simulink model "mu_t_2021b_temp"  (R2023b)
settings: Solver=VariableStepAuto  StartTime=0.0  StopTime=120  FixedStep=0.01  RelTol=1e-3
InitFcn:
  | %rho_0t=[0.29;0.29;0.29]; %m
  | %V_0t=[-0.001;-0.001;0];%[-0.0005;-0.0005;0];
  | %w_t=[0;0;-0.002];
  | 
  | 
  | %rho_0t=[0.3;0.3;0.2]; %m
  | %V_0t=[-0.001;-0.001;0];%[-0.0005;-0.0005;0];
  | %w_t=[0;0;-0.001];
values from neighbouring files (symbols this model uses):
  g_cm = zeros(4,4,n)    [Initiate_KUKA_inv.m]    (also in KUKA_Main.m)
  iota0 = eye(6,6)    [Initiate_KUKA_inv.m]    (also in KUKA_Main.m)
  K_d = 10*[1.3*eye(3) zeros(3);zeros(3) 0.8*eye(3)]    [Initiate_FQ.m]    (also in Initiate_KUKA_inv.m = 5*[0.7*eye(3) zeros(3);zeros(3) 0.5*eye(3)]; KUKA_Main.m = 50*[0.7*eye(3) zeros(3);zeros(3) 0.5*eye(3)])
  K_i = 5*[0.1*eye(3) zeros(3);zeros(3) 0.01*eye(3)]    [Initiate_FQ.m]    (also in Initiate_KUKA_inv.m = 5*[0.01*eye(3) zeros(3);zeros(3) 0.001*eye(3)]; KUKA_Main.m = 50*[0.01*eye(3) zeros(3);zeros(3) 0.001*eye(3)])
  K_p = 100*[0.1 0 0 0 0 0;0 0.1 0 0 0 0; 0 0 0.1 0 0 0; 0 0 0 0.01 0 0 ... (first row only)    [Initiate_FQ.m]    (also in Initiate_KUKA_inv.m = 5*[0.1 0 0 0 0 0;0 0.1 0 0 0 0; 0 0 0.1 0 0 0; 0 0 0 0.01 0 ; KUKA_Main.m = 50*[0.1 0 0 0 0 0;0 0.1 0 0 0 0; 0 0 0.1 0 0 0; 0 0 0 0.01 0)
  K_w = 200*eye(7)    [Initiate_FQ.m]
  K_wd = 2*eye(7)    [Initiate_FQ.m]
  M0 = M_temp.M0.data(:,:,1)    [Initiate_FQ.m]    (also in KUKA_Main.m)
  m0 = robot.Bodies{1,n+1}.Mass    [Initiate_KUKA_inv.m]    (also in KUKA_Main.m)
  m0_frak = diag_M(1:6,1:6)    [Initiate_KUKA_inv.m]
  M0m = M_temp.M0m.data(:,:,1)    [Initiate_FQ.m]    (also in KUKA_Main.m)
  m_diag = diag_M(7:end,7:end)    [Initiate_KUKA_inv.m]
  M_t = (((Adjoint(g_It))'\M_t_body)/(Adjoint(g_It)))    [Initiate_FQ.m]    (also in Initiate_KUKA_inv.m = [eye(3)*mt zeros(3); zeros(3) eye(3)*80]; KUKA_Main.m = [eye(3)*mt zeros(3); zeros(3) eye(3)*80])
  Mm = simplify(transpose(Xi_m)*transpose(Lm)*diagM*Lm*Xi_m)    [KUKA_Main.m]
  mm = zeros(1,n)    [Initiate_KUKA_inv.m]    (also in KUKA_Main.m)
  mu = P0    [Initiate_FQ.m]    (also in Initiate_KUKA_inv.m = zeros(6,1); KUKA_Main.m = P)
  mu_t = inv((Adjoint(g_It))')*M_t_body*[V_It;w_t]    [Initiate_FQ.m]    (also in Initiate_KUKA_inv.m = M_t*[V_0t;w_t]; KUKA_Main.m = M_t*[V_0t;w_t])
  q_dot_m = [0;0;0;0;0;0;0]    [Initiate_FQ.m]    (also in Initiate_KUKA_inv.m; KUKA_Main.m = [qdot1;qdot2;qdot3;qdot4;qdot5;qdot6;qdot7])
  q_m = [0.2;1.2;0.3;2.5;0.5;1.5;0.6]    [Initiate_FQ.m]    (also in Initiate_KUKA_inv.m = [0;0;0;0;0;0;0]; KUKA_Main.m = [q_m1;q_m2;q_m3;q_m4;q_m5;q_m6;q_m7])
  rho_It = [-0.3;-0.3;-0.1]    [Initiate_FQ.m]
  sc_size = 1    [Initiate_KUKA_inv.m]    (also in KUKA_Main.m)
  V_I0 = [-0.0001;-0.0001;0.0;-0.001;0.001;0.002]    [Initiate_FQ.m]    (also in Initiate_KUKA_inv.m = [0;0;0;0;0;0]; KUKA_Main.m = [0;0;0;0;0;0])
  V_It = 0.1.*[0.01;0.01;0]    [Initiate_FQ.m]
  Xi_m = Xi_m(1:robot.n*6,1:robot.n)    [KUKA_Main.m]
  Xi_m_matrix = zeros(6*n,n)    [Initiate_KUKA_inv.m]    (also in KUKA_Main.m)
undefined symbols (not defined in the file or in its folder): Dt, Dt_s, g_cm0, g_It00, I0, Ie, Im, me, noise_st, X, Y, Z
libraries: nesl_utility x195, sm_lib x180, robotcorelib x12, simulink x6
(part 1 of 8)
settings Model: Creator=Bmmog  LastModifiedBy=Bmmog
settings SolverCC: ZeroCrossAlgorithm=Adaptive
settings DataIOCC: ReturnWorkspaceOutputsName=tp1ae71780_9f9b_41fc_80d6_93119145c185
settings DebuggingCC: UnconnectedInputMsg=warning  UnconnectedOutputMsg=warning  UnconnectedLineMsg=warning
settings ModelReferenceCC: EnableRefExpFcnMdlSchedulingChecks=on
settings RTWCC: DLArmComputeVersion=19.05
settings ExplorerConfigSet: InternalSimMechanicsExplorerSettings="<ExplorerConfiguration><canonicalview>default</canonicalview><AnimationSetting><BasePlaybackSpeed>1.0</BasePlaybackSpeed><PlaybackSpeedFactor>1.0</PlaybackSpeedFactor></AnimationSetting><TilePanel><TileInfo><Tiles Columns=\"1\" Count=\"1\" Rows=\"1\"><Column Weight=\"1\"/><Row Weight=\"1\"/><Tile Height=\"1\" Width=\"1\" X=\"0\" Y=\"0\"/></Tiles></TileInfo><SceneInfo><SceneViewer><BGColor><R>0.60000002384185791</R><G>0.60000002384185791</G><B>0.60000002384185791</B></BGColor><Camera><DoPerspective>off</DoPerspective><Position><X>0.589775080981291833</X><Y>-1.46493128404912909</Y><Z>0.784080153206962893</Z></Position><Center><X>-0.149105792545367294</X><Y>0.231974603355053599</Y><Z>-0.0696143327165401893</Z></Center><Up><X>0.0771327039681207333</X><Y>0.474680075340175867</Y><Z>0.876772132343182631</Z></Up><ViewLimDist>1</ViewLimDist><YLim>0.0938244390560590141</YLim><XLim>0.109167654126007874</XLim></Camera></SceneViewer></SceneInfo></TilePanel><MechEditorPanel><Cameras/><GfxPanelCameraMap/><VideoCreator><PlaybackSpeedRatio>1.0</PlaybackSpeedRatio><FrameRate>30</FrameRate><VideoFormat>Motion JPEG AVI</VideoFormat><FrameSize>auto</FrameSize></VideoCreator></MechEditorPanel></ExplorerConfiguration>"

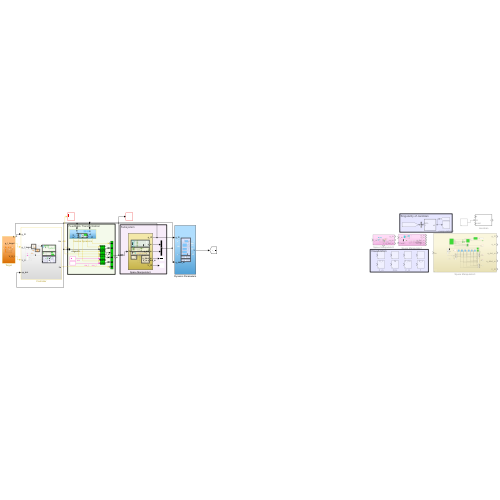
[thumbnail: Simulink's stored preview of the top-level diagram]
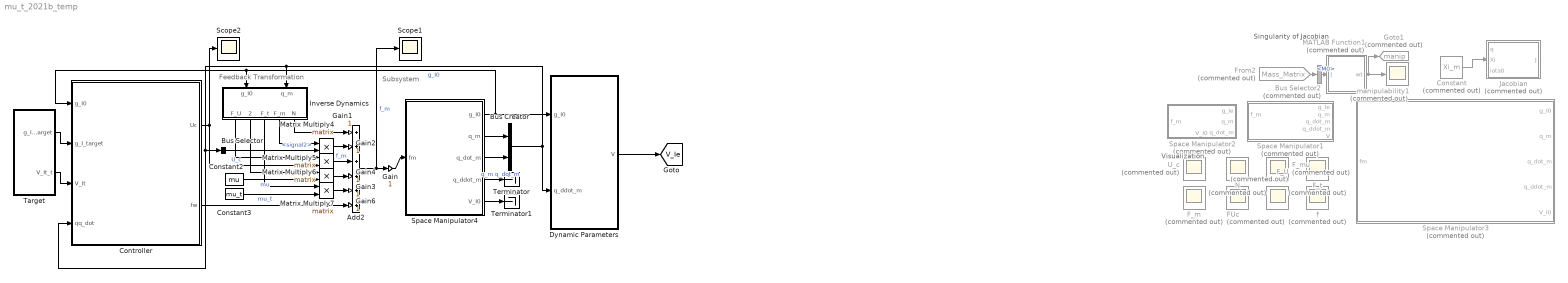
== system mu_t_2021b_temp ==
  note: Subsystem
  note: Feedback Transformation
  note: Singularity of Jacobian
  note: Visualization
  Add2 : Sum  Inputs=++++++
  Bus Creator : BusCreator  Inputs=2
  Bus Selector : BusSelector  OutputSignals=signal2
  Bus Selector2 : BusSelector  Commented=on  OutputSignals=M0
  Constant : Constant  Commented=on  Value=Xi_m
  Constant2 : Constant  Value=mu
  Constant3 : Constant  Value=mu_t
  Controller : Subsystem
  Dynamic Parameters : Subsystem
  FUc : Scope  Commented=on
  F_U : Scope  Commented=on
  F_m : Scope  Commented=on
  F_mu : Scope  Commented=on
  F_t : Scope  Commented=on
  From2 : From  Commented=on  GotoTag=Mass_Matrix  TagVisibility=global
  Gain{,1..4,6} (6 alike) : Gain
  Goto1 : Goto  Commented=on  GotoTag=manip  TagVisibility=global
  Inverse Dynamics : Subsystem
  Jacobian : MATLAB Function  Commented=on  TreatAsAtomicUnit=on
  MATLAB Function1 : MATLAB Function  Commented=on  TreatAsAtomicUnit=on
  Matrix Multiply{4..7} (4 alike) : Product  Multiplication=Matrix(*)
  N : Scope  Commented=on
  Scope1 : Scope
  Scope2 : Scope
  Space Manipulator1 : Subsystem  Commented=on
  Space Manipulator2 : Subsystem  Commented=on
      settings: PortSchema="{\"entries\":[{\"content\":{\"sides\":[{\"content\":{\"connectorIds\":[\"In1\"]},\"type\":\"ConnectorPlacement.EquallySpacedRectSide\",\"uuid\":\"530c21f8-fd54-4a84-9ce8-3a95f84fd0bc\"},{\"content\":{\"connectorIds\":[\"Out1\",\"Out2\",\"Out3\"],\"side\":\"RIGHT\"},\"type\":\"ConnectorPlacement.EquallySpacedRectSide\",\"uuid\":\"3d1ca3bb-457e-45f0-8a55-d4d08374b273\"},{\"content\":{\"connectorIds\":[],\"side\":\"TOP\"},\"type\":\"ConnectorPlacement.EquallySpacedRectSide\",\"uuid\":\"24d553c5-4913-4f02-8b85-43cdd650a04b\"},{\"content\":{\"connectorIds\":[\"Out4\"],\"side\":\"BOTTOM\"},\"type\":\"ConnectorPlacement.EquallySpacedRectSide\",\"uuid\":\"b0ec554d-8dce-4af2-8e04-261e5fffea9f\"}]},\"type\":\"ConnectorPlacement.EquallySpacedConnector\",\"uuid\":\"032cf2d7-4a61-467d-a02b-78dcb243a1bb\"}],\"packageUris\":[\"http://schema.mathworks.com/mf0/Connector/R2020b\"],\"version\":\"1.0\"}"
  Space Manipulator3 : Subsystem  Commented=on
  Space Manipulator4 : Subsystem
  Target : Subsystem
  Terminator : Terminator
  Terminator1 : Terminator
  U_c : Scope  Commented=on
  f : Scope  Commented=on
  manipulability1 : Scope  Commented=on
  tag scope: V_Ie=global
  wires:
  Target/2(V_It_t) -> Controller/3(V_It)
  Space Manipulator4/1(g_I0) -> Inverse Dynamics/1(g_I0), Controller/1(g_I0), Dynamic Parameters/1(g_I0)  "g_I0"
  Inverse Dynamics/3(F_t) -> Matrix Multiply7/1
  Matrix Multiply5/1 -> Add2/3  "f_m"
  Inverse Dynamics/2(F_mu) -> Matrix Multiply6/1
  Inverse Dynamics/4(F_m) -> Matrix Multiply4/1
  Constant3/1 -> Matrix Multiply7/2  "mu_t"
  Constant2/1 -> Matrix Multiply6/2  "mu"
  Bus Creator/1 -> Inverse Dynamics/2("q_m "), Bus Selector/1, Controller/4(qq_dot), Dynamic Parameters/2(q_ddot_m)
  Bus Selector/1 -> Matrix Multiply4/2  "<signal2>"
  Space Manipulator4/4(q_ddot_m) -> Terminator/1  "q_m q_dot_m"
  Gain/1 -> Space Manipulator4/1(fm)
  Target/1(g_I_target) -> Controller/2(g_I_target)
  Add2/1 -> Scope1/1, Gain/1  "f_m"
  Gain1/1 -> Add2/1
  Gain2/1 -> Add2/2
  Gain3/1 -> Add2/5
  Gain4/1 -> Add2/4
  Controller/1(Uc) -> Scope2/1, Matrix Multiply5/2  "U_c"
  Inverse Dynamics/1(F_U) -> Matrix Multiply5/1
  Matrix Multiply4/1 -> Gain2/1
  Matrix Multiply6/1 -> Gain4/1
  Inverse Dynamics/5(N) -> Gain1/1
  Matrix Multiply7/1 -> Gain3/1
  Space Manipulator4/2(q_m) -> Bus Creator/1
  Space Manipulator4/3(q_dot_m) -> Bus Creator/2
  Space Manipulator4/5(V_I0) -> Terminator1/1
  Constant/1 -> Jacobian/2(Xi)
  From2/1 -> Bus Selector2/1
  Bus Selector2/1 -> MATLAB Function1/1(J)  "<M0>"
  Gain6/1 -> Add2/6
  MATLAB Function1/1(wt) -> Goto1/1, manipulability1/1
  Controller/2(fw) -> Gain6/1
  Dynamic Parameters/1(V) -> [V_Ie]

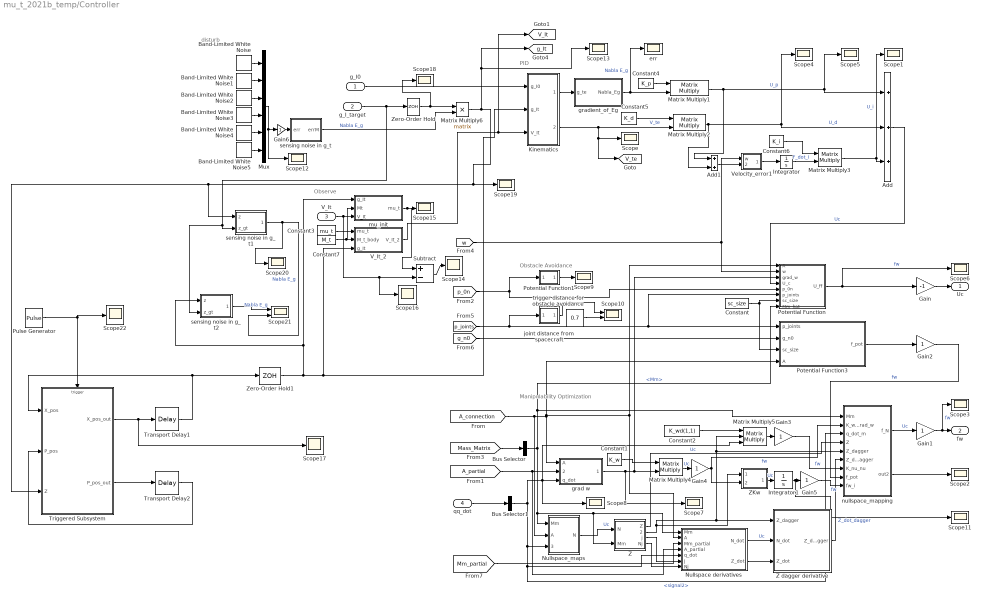
== system mu_t_2021b_temp/Controller ==
  note: PID
  note: Manipulability Optimization
  note: Obstacle Avoidance
  note: Observe
  note: disturb
  g_I0 : Inport
  g_I_target : Inport  Port=2
  V_It : Inport  Port=3
  qq_dot : Inport  Port=4
  Add : Sum  Inputs=+++
  Add1 : Sum
  Band-Limited White Noise : simulink/Sources/Band-Limited White Noise  Cov=[noise_st]  Ts=Dt_s  seed=[23341]
  Band-Limited White Noise1 : simulink/Sources/Band-Limited White Noise  Cov=[noise_st]  Ts=Dt_s  seed=[23342]
  Band-Limited White Noise2 : simulink/Sources/Band-Limited White Noise  Cov=[noise_st]  Ts=Dt_s  seed=[23343]
  Band-Limited White Noise3 : simulink/Sources/Band-Limited White Noise  Cov=[noise_st]  Ts=Dt_s  seed=[23344]
  Band-Limited White Noise4 : simulink/Sources/Band-Limited White Noise  Cov=[noise_st]  Ts=Dt_s  seed=[23345]
  Band-Limited White Noise5 : simulink/Sources/Band-Limited White Noise  Cov=[noise_st]  Ts=Dt_s  seed=[23346]
  Bus Selector : BusSelector  OutputSignals=Mm
  Bus Selector1 : BusSelector  OutputSignals=signal2
  Constant : Constant  Value=sc_size
  Constant1 : Constant  Value=K_w
  Constant2 : Constant  Value=K_wd(1,1)
  Constant3 : Constant  Value=mu_t
  Constant4 : Constant  Value=K_p
  Constant5 : Constant  Value=K_d
  Constant6 : Constant  Value=K_i
  Constant7 : Constant  Value=M_t
  Gain : Gain  Gain=-1
  Gain{1..6} (6 alike) : Gain
  Integrator : Integrator
  Integrator1 : Integrator
  Kinematics : Subsystem
  Matrix Multiply{1..4,6} (5 alike) : Product  Multiplication=Matrix(*)
  Matrix Multiply5 : Product  Inputs=3  Multiplication=Matrix(*)
  Mux : Mux  Inputs=6
  Nullspace derivatives : MATLAB Function  TreatAsAtomicUnit=on
  Nullspace_maps : MATLAB Function  TreatAsAtomicUnit=on
  Potential Function : MATLAB Function  TreatAsAtomicUnit=on
  Potential Function1 : MATLAB Function  TreatAsAtomicUnit=on
  Potential Function3 : MATLAB Function  TreatAsAtomicUnit=on
  Pulse Generator : DiscretePulseGenerator  PulseType=Time based  Period=Dt  PulseWidth=10
  Scope{,1..9,11..20,22} (21 alike) : Scope
  Scope10 : Scope  NumInputPorts=2
  Scope21 : Scope  NumInputPorts=2
  Subtract : Sum  Inputs=+-
  Transport Delay1 : TransportDelay  DelayTime=Dt  InitialOutput=g_It00  TransDelayFeedthrough=on
  Transport Delay2 : TransportDelay  DelayTime=Dt  InitialOutput=zeros(6)  TransDelayFeedthrough=on
  Triggered Subsystem : Subsystem  TreatAsAtomicUnit=on
  V_It_2 : MATLAB Function  TreatAsAtomicUnit=on
  Velocity_error1 : MATLAB Function  TreatAsAtomicUnit=on
  Z : MATLAB Function  TreatAsAtomicUnit=on
  Z dagger derivative : MATLAB Function  TreatAsAtomicUnit=on
  ZKw : MATLAB Function  TreatAsAtomicUnit=on
  Zero-Order Hold : ZeroOrderHold  SampleTime=Dt_s
  Zero-Order Hold1 : ZeroOrderHold  SampleTime=Dt
  err : Scope
  grad w : MATLAB Function  TreatAsAtomicUnit=on
  gradient_of_Eg : MATLAB Function  TreatAsAtomicUnit=on
  joint distance from spacecraft : MATLAB Function  TreatAsAtomicUnit=on
  mu_init : MATLAB Function  TreatAsAtomicUnit=on
  nullspace_mapping : MATLAB Function  TreatAsAtomicUnit=on
  sensing noise in g_t : MATLAB Function  TreatAsAtomicUnit=on
  sensing noise in g_t1 : MATLAB Function  TreatAsAtomicUnit=on
  sensing noise in g_t2 : MATLAB Function  TreatAsAtomicUnit=on
  trigger distance for obstacle avoidance : Constant  Value=0.7
  Uc : Outport
  fw : Outport  Port=2
  tag scope: V_It=global, V_te=global, g_It=global
  wires:
  [A_connection] -> Nullspace_maps/2(A), Potential Function3/4(A), Nullspace derivatives/2(A), Potential Function/1(A), grad w/1(A)
  [A_partial] -> Nullspace derivatives/4(A_partial), grad w/2(A_partial)
  qq_dot/1 -> Bus Selector1/1
  [Mass_Matrix] -> Bus Selector/1
  Bus Selector/1 -> Nullspace_maps/1(Mm), Z/2(Mm), Nullspace derivatives/1(Mm), Potential Function/8(Mm_hat), nullspace_mapping/1(Mm)  "<Mm>"
  Gain/1 -> Uc/1
  g_I0/1 -> Kinematics/1(g_I0)
  Add/1 -> Potential Function/4(U_c)  "Uc"
  Kinematics/1(g_te1) -> gradient_of_Eg/1(g_te)
  Add1/1 -> Velocity_error1/2(in)
  Matrix Multiply2/1 -> Scope4/1, Add/2, Add1/2  "U_d"
  gradient_of_Eg/1(Nabla_Eg) -> err/1, Matrix Multiply1/2  "Nabla E_g"
  Constant4/1 -> Matrix Multiply1/1
  Kinematics/2(V_te) -> [V_te], Scope/1, Matrix Multiply2/2  "V_te"
  Constant6/1 -> Matrix Multiply3/1
  Integrator/1 -> Matrix Multiply3/2  "F_dot_I"
  Matrix Multiply1/1 -> Scope5/1, Add/1, Add1/1  "U_p"
  Constant5/1 -> Matrix Multiply2/1
  Bus Selector1/1 -> Scope8/1, grad w/3(q_dot), Matrix Multiply5/3, nullspace_mapping/3(q_dot_m), Nullspace derivatives/5(q_dot), Nullspace_maps/3(q_dot_m)  "<signal2>"
  Gain1/1 -> fw/1, Scope3/1  "fw"
  Constant1/1 -> Matrix Multiply4/1
  grad w/1(grad_w) -> Scope7/1, Potential Function/3(grad_w), Matrix Multiply4/2
  Matrix Multiply5/1 -> Gain3/1
  Constant2/1 -> Matrix Multiply5/1
  Matrix Multiply4/1 -> Gain4/1  "Uc"
  Matrix Multiply3/1 -> Scope1/1, Add/3  "U_i"
  nullspace_mapping/1(f_N) -> Gain1/1  "Uc"
  [w] -> Potential Function/2(w), Velocity_error1/1(w)
  Potential Function/1(U_ff) -> Gain/1, Scope6/1  "fw"
  Velocity_error1/1(out) -> Integrator/1
  [p_0n] -> Potential Function1/1(p_0n), Potential Function/5(p_0n)
  Potential Function1/1(w_p) -> Scope9/1
  [p_joints] -> joint distance from spacecraft/1(p_joints), Potential Function/6(p_joints), Potential Function3/1(p_joints)
  joint distance from spacecraft/1(pnorm) -> Scope10/1
  [g_n0] -> Potential Function3/2(g_n0)
  Potential Function3/1(f_pot) -> Gain2/1
  Constant/1 -> Potential Function3/3(sc_size), Potential Function/7(sc_size)
  trigger distance for obstacle avoidance/1 -> Scope10/2
  Gain3/1 -> nullspace_mapping/7(K_nu_nu)  "fw"
  Nullspace derivatives/1(N_dot) -> Z dagger derivative/2(N_dot)  "Uc"
  Nullspace derivatives/2(Z_dot) -> Z dagger derivative/3(Z_dot)
  Z dagger derivative/1(Z_dot_dagger) -> nullspace_mapping/6(Z_dot_dagger)  "Z_dot_dagger"
  Nullspace_maps/1(N) -> Z/1(N)  "Uc"
  [Mm_partial] -> Nullspace derivatives/3(Mm_partial)
  Z/1(Z) -> nullspace_mapping/4(Z)  "Uc"
  Gain4/1 -> ZKw/2(K_w_grad_w), nullspace_mapping/2(K_w_grad_w)  "fw"
  nullspace_mapping/2(out2) -> Scope2/1
  Z/2(Z_dagger) -> ZKw/1(Z_dagger), nullspace_mapping/5(Z_dagger), Matrix Multiply5/2, Z dagger derivative/1(Z_dagger)
  ZKw/1(out) -> Integrator1/1  "Uc"
  Integrator1/1 -> Scope11/1, Gain5/1
  Gain5/1 -> nullspace_mapping/9(fw_i)  "fw"
  V_It/1 -> mu_init/3(V_It), Scope16/1, Subtract/2
  Constant3/1 -> V_It_2/1(mu_t)
  mu_init/1(mu_t) -> Subtract/1, Scope15/1
  Constant7/1 -> mu_init/2(Mt), V_It_2/2(M_t_body)
  Gain2/1 -> nullspace_mapping/8(f_pot)  "fw"
  Band-Limited White Noise/1 -> Mux/1
  sensing noise in g_t/1(errM) -> Matrix Multiply6/2  "Nabla E_g"
  Band-Limited White Noise2/1 -> Mux/3
  Band-Limited White Noise4/1 -> Mux/5
  Band-Limited White Noise3/1 -> Mux/4
  Band-Limited White Noise1/1 -> Mux/2
  Zero-Order Hold/1 -> Scope18/1, Matrix Multiply6/1
  Z/3(j) -> Nullspace derivatives/6(j)
  Z/4(Nj) -> Nullspace derivatives/7(Nj)
  Gain6/1 -> sensing noise in g_t/1(err)
  V_It_2/1(V_It_2) -> Kinematics/3(V_It), [V_It]
  Subtract/1 -> Scope14/1
  Matrix Multiply6/1 -> sensing noise in g_t1/1(z), Triggered Subsystem/3(Z), Scope19/1, [g_It], Scope13/1
  g_I_target/1 -> sensing noise in g_t2/2(z_gt), sensing noise in g_t1/2(z_gt), Zero-Order Hold/1
  sensing noise in g_t2/1(errM) -> Scope21/1  "Nabla E_g"
  Triggered Subsystem/1(X_pos_out) -> Scope17/1, Transport Delay1/1
  Transport Delay1/1 -> Triggered Subsystem/1(X_pos), Zero-Order Hold1/1
  Triggered Subsystem/2(P_pos_out) -> Transport Delay2/1
  Transport Delay2/1 -> Triggered Subsystem/2(P_pos)
  Mux/1 -> Scope12/1, Gain6/1
  Band-Limited White Noise5/1 -> Mux/6
  Pulse Generator/1 -> Triggered Subsystem/Trigger, Scope22/1
  Zero-Order Hold1/1 -> Kinematics/2(g_It), V_It_2/3(g_It), sensing noise in g_t2/1(z), mu_init/1(g_It)
  sensing noise in g_t1/1(errM) -> Scope20/1, Scope21/2  "Nabla E_g"

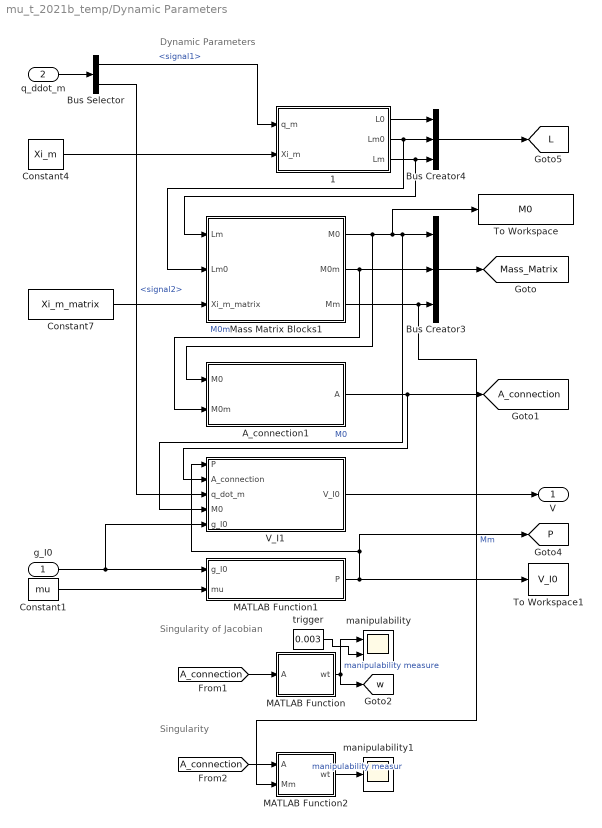
== system mu_t_2021b_temp/Dynamic Parameters ==
  note: Singularity of Jacobian
  note: Dynamic Parameters
  note: Singularity
  g_I0 : Inport
  q_ddot_m : Inport  Port=2
  " 1" : MATLAB Function  TreatAsAtomicUnit=on
  A_connection1 : Subsystem
  Bus Creator3 : BusCreator  Inputs=M0,M0m,Mm
  Bus Creator4 : BusCreator  Inputs=3
  Bus Selector : BusSelector  OutputSignals=signal1,signal2
  Constant1 : Constant  Value=mu
  Constant4 : Constant  Value=Xi_m
  Constant7 : Constant  Value=Xi_m_matrix
  MATLAB Function : MATLAB Function  TreatAsAtomicUnit=on
  MATLAB Function1 : MATLAB Function  TreatAsAtomicUnit=on
  MATLAB Function2 : MATLAB Function  TreatAsAtomicUnit=on
  Mass Matrix Blocks1 : Subsystem
  To Workspace : ToWorkspace  VariableName=M0  SaveFormat=Timeseries  SampleTime=-1
  To Workspace1 : ToWorkspace  VariableName=V_I0  SaveFormat=Timeseries  SampleTime=-1
  V_I1 : MATLAB Function  TreatAsAtomicUnit=on
  manipulability : Scope  NumInputPorts=2
  manipulability1 : Scope
  trigger : Constant  Value=0.003
  V : Outport
  tag scope: A_connection=global, L=global, Mass_Matrix=global, P=global, w=global
  wires:
  MATLAB Function1/1(P) -> To Workspace1/1, [P], V_I1/1(P)
  Constant1/1 -> MATLAB Function1/2(mu)
  g_I0/1 -> V_I1/5(g_I0), MATLAB Function1/1(g_I0)
  A_connection1/1(A) -> [A_connection], V_I1/2(A_connection)
  Mass Matrix Blocks1/1(M0) -> A_connection1/1(M0), To Workspace/1, V_I1/4(M0), Bus Creator3/1  "M0"
  V_I1/1(V_I0) -> V/1
  Mass Matrix Blocks1/3(Mm) -> MATLAB Function2/2(Mm), Bus Creator3/3  "Mm"
  Bus Creator3/1 -> [Mass_Matrix]
  Bus Creator4/1 -> [L]
  q_ddot_m/1 -> Bus Selector/1
  " 1"/2(Lm0) -> Mass Matrix Blocks1/2(Lm0), Bus Creator4/2
  " 1"/1(L0) -> Bus Creator4/1
  Constant4/1 -> " 1"/2(Xi_m)
  " 1"/3(Lm) -> Bus Creator4/3, Mass Matrix Blocks1/1(Lm)
  Constant7/1 -> Mass Matrix Blocks1/3(Xi_m_matrix)
  Mass Matrix Blocks1/2(M0m) -> Bus Creator3/2, A_connection1/2(M0m)  "M0m"
  Bus Selector/2 -> V_I1/3(q_dot_m)  "<signal2>"
  Bus Selector/1 -> " 1"/1(q_m)  "<signal1>"
  MATLAB Function/1(wt) -> [w], manipulability/1  "manipulability measure"
  [A_connection] -> MATLAB Function/1(A)
  trigger/1 -> manipulability/2
  [A_connection] -> MATLAB Function2/1(A)
  MATLAB Function2/1(wt) -> manipulability1/1  "manipulability measur"

== system mu_t_2021b_temp/Inverse Dynamics ==
  note: f_m
  g_I0 : Inport
  "q_m " : Inport  Port=2
  A_dot : MATLAB Function  TreatAsAtomicUnit=on
  Bus Selector : BusSelector  OutputSignals=M0,Mm
  Bus Selector2 : BusSelector  OutputSignals=signal1,signal2
  C_hat : Subsystem  Commented=on
  C_hat1 : Subsystem
  Inverse Dynamics : Subsystem
  M0_dot : MATLAB Function  TreatAsAtomicUnit=on
  N_hat : Subsystem  Commented=on
  N_hat1 : Subsystem
  F_U : Outport
  F_mu : Outport  Port=2
  F_t : Outport  Port=3
  F_m : Outport  Port=4
  N : Outport  Port=5
  wires:
  [P] -> N_hat1/4(P)
  [Mass_Matrix] -> Bus Selector/1
  Bus Selector/1 -> N_hat1/5(M0), Inverse Dynamics/2(<M0>)  "<M0>"
  g_I0/1 -> Inverse Dynamics/1(g_I0)
  Inverse Dynamics/1(F_U) -> F_U/1
  Inverse Dynamics/2(F_mu) -> F_mu/1
  Inverse Dynamics/3(F_t) -> F_t/1
  Inverse Dynamics/4(F_m) -> F_m/1
  Bus Selector/2 -> Inverse Dynamics/3(Mm)  "<Mm>"
  Bus Selector2/1 -> N_hat1/1(q_m), C_hat1/1(q_m)  "<signal1>"
  Bus Selector2/2 -> A_dot/2(q_m_dot), M0_dot/2(q_m_dot), N_hat1/2(q_dot_m), C_hat1/2(q_dot_m)  "<signal2>"
  C_hat1/1(M0_partial) -> M0_dot/1(M0_partial)
  C_hat1/2(Out1) -> A_dot/1(A_partial)
  C_hat1/3(C_hat1) -> Inverse Dynamics/6(C_hat)
  M0_dot/1(M0_dot) -> Inverse Dynamics/4(M0_dot)
  A_dot/1(A_dot) -> Inverse Dynamics/5(A_dot)
  "q_m "/1 -> Bus Selector2/1
  [A_connection] -> N_hat1/3(A)
  N_hat1/1(N_hat1) -> N/1

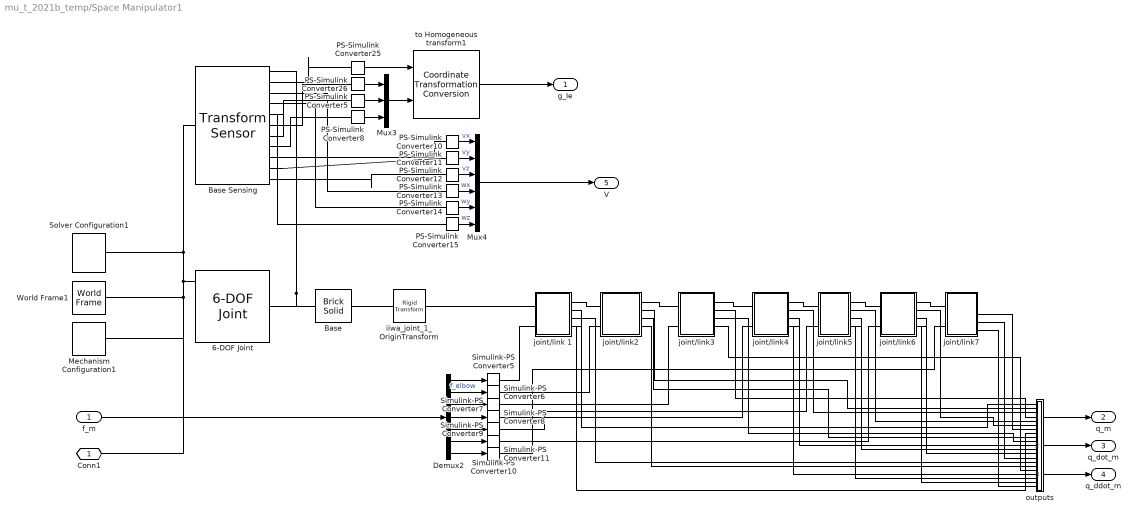
== system mu_t_2021b_temp/Space Manipulator1 ==
  f_m : Inport
  6-DOF Joint : sm_lib/Joints/6-DOF Joint  JointMode=Normal  SenseConstraintForce=off  SenseConstraintForceX=off  SenseConstraintForceY=off  SenseConstraintForceZ=off  SenseConstraintTorque=off  SenseConstraintTorqueX=off  SenseConstraintTorqueY=off  SenseConstraintTorqueZ=off  SenseTotalForce=off  SenseTotalForceX=off  SenseTotalForceY=off  SenseTotalForceZ=off  SenseTotalTorque=off  SenseTotalTorqueX=off  SenseTotalTorqueY=off  SenseTotalTorqueZ=off  CompositeWrenchDir=FollowerOnBase  CompositeWrenchFrame=BaseFrame  PxEquilibriumPosition=0  PxEquilibriumPositionUnits=m  PxSpringStiffness=0  PxSpringStiffnessUnits=N/m  PxDampingCoefficient=0  PxDampingCoefficientUnits=N/(m/s)  PxTorqueActuationMode=InputTorque  PxMotionActuationMode=ComputedMotion  PxSensePosition=off  PxSenseVelocity=off  PxSenseAcceleration=off  PxSenseTorqueForce=off  PxSenseLowerLimitTorqueForce=off  PxSenseUpperLimitTorqueForce=off  PxLowerLimitSpecify=off  PxLowerLimitBound=-1  PxLowerLimitBoundUnits=m  PxLowerLimitStiffness=1e6  PxLowerLimitStiffnessUnits=N/m  PxLowerLimitDamping=1e3  PxLowerLimitDampingUnits=N/(m/s)  PxLowerLimitTransitionRegionWidth=1e-4  PxLowerLimitTransitionRegionWidthUnits=m  PxUpperLimitSpecify=off  PxUpperLimitBound=1  PxUpperLimitBoundUnits=m  PxUpperLimitStiffness=1e6  PxUpperLimitStiffnessUnits=N/m  PxUpperLimitDamping=1e3  PxUpperLimitDampingUnits=N/(m/s)  PxUpperLimitTransitionRegionWidth=1e-4  PxUpperLimitTransitionRegionWidthUnits=m  PxPositionTargetSpecify=off  PxPositionTargetPriority=High  PxPositionTargetValue=0  PxPositionTargetValueUnits=m  PxVelocityTargetSpecify=on  PxVelocityTargetPriority=High  PxVelocityTargetValue=V_I0(1)  PxVelocityTargetValueUnits=m/s  PyEquilibriumPosition=0  PyEquilibriumPositionUnits=m  PySpringStiffness=0  PySpringStiffnessUnits=N/m  PyDampingCoefficient=0  PyDampingCoefficientUnits=N/(m/s)  PyTorqueActuationMode=InputTorque  PyMotionActuationMode=ComputedMotion  PySensePosition=off  PySenseVelocity=off  PySenseAcceleration=off  PySenseTorqueForce=off  PySenseLowerLimitTorqueForce=off  PySenseUpperLimitTorqueForce=off  PyLowerLimitSpecify=off  PyLowerLimitBound=-1  PyLowerLimitBoundUnits=m  PyLowerLimitStiffness=1e6  PyLowerLimitStiffnessUnits=N/m  PyLowerLimitDamping=1e3  PyLowerLimitDampingUnits=N/(m/s)  PyLowerLimitTransitionRegionWidth=1e-4  PyLowerLimitTransitionRegionWidthUnits=m  PyUpperLimitSpecify=off  PyUpperLimitBound=1  PyUpperLimitBoundUnits=m  PyUpperLimitStiffness=1e6  PyUpperLimitStiffnessUnits=N/m  PyUpperLimitDamping=1e3  PyUpperLimitDampingUnits=N/(m/s)  PyUpperLimitTransitionRegionWidth=1e-4  PyUpperLimitTransitionRegionWidthUnits=m  PyPositionTargetSpecify=off  PyPositionTargetPriority=High  PyPositionTargetValue=0  PyPositionTargetValueUnits=m  PyVelocityTargetSpecify=on  PyVelocityTargetPriority=High  PyVelocityTargetValue=V_I0(2)  PyVelocityTargetValueUnits=m/s  PzEquilibriumPosition=0  PzEquilibriumPositionUnits=m  PzSpringStiffness=0  PzSpringStiffnessUnits=N/m  PzDampingCoefficient=0  PzDampingCoefficientUnits=N/(m/s)  PzTorqueActuationMode=InputTorque  PzMotionActuationMode=ComputedMotion  PzSensePosition=off  PzSenseVelocity=off  PzSenseAcceleration=off  PzSenseTorqueForce=off  PzSenseLowerLimitTorqueForce=off  PzSenseUpperLimitTorqueForce=off  PzLowerLimitSpecify=off  PzLowerLimitBound=-1  PzLowerLimitBoundUnits=m  PzLowerLimitStiffness=1e6  PzLowerLimitStiffnessUnits=N/m  PzLowerLimitDamping=1e3  PzLowerLimitDampingUnits=N/(m/s)  PzLowerLimitTransitionRegionWidth=1e-4  PzLowerLimitTransitionRegionWidthUnits=m  PzUpperLimitSpecify=off  PzUpperLimitBound=1  PzUpperLimitBoundUnits=m  PzUpperLimitStiffness=1e6  PzUpperLimitStiffnessUnits=N/m  PzUpperLimitDamping=1e3  PzUpperLimitDampingUnits=N/(m/s)  PzUpperLimitTransitionRegionWidth=1e-4  PzUpperLimitTransitionRegionWidthUnits=m  PzPositionTargetSpecify=off  PzPositionTargetPriority=High  PzPositionTargetValue=0  PzPositionTargetValueUnits=m  PzVelocityTargetSpecify=on  PzVelocityTargetPriority=High  PzVelocityTargetValue=V_I0(3)  PzVelocityTargetValueUnits=m/s  SphEqPosRotationMethod=None  SphEqPosRotationAngleUnits=deg  SphEqPosRotationStandardAxis=+Z  SphEqPosRotationAngle=0.0  SphEqPosRotationArbitraryAxis=[0 0 1]  SphEqPosFollAlignAxisA=+X  SphEqPosBaseAlignAxisA=+Y  SphEqPosFollAlignAxisB=+Y  SphEqPosBaseAlignAxisB=+Z  SphEqPosRotationSequenceAxes=FollowerAxes  SphEqPosRotationSequence=XYX  SphEqPosRotationSequenceAngles=[0 0 0]  SphEqPosRotationSequenceAnglesUnits=deg  SphEqPosRotationMatrix=[1 0 0; 0 1 0; 0 0 1]  SphEqPosQuaternion=[1 0 0 0]  SphSpringStiffness=0  SphSpringStiffnessUnits=N*m/deg  SphDampingCoefficient=0  SphDampingCoefficientUnits=N*m/(deg/s)  SphActuateTorqueX=off  SphActuateTorqueY=off  SphActuateTorqueZ=off  SphActuateTorque=off  SphTorqueActuationMode=NoTorque  SphMotionActuationMode=ComputedMotion  SphActuationFrame=BaseFrame  SphSensePosition=off  SphSenseVelocityX=off  SphSenseVelocityY=off  SphSenseVelocityZ=off  SphSenseVelocity=off  SphSenseAccelerationX=off  SphSenseAccelerationY=off  SphSenseAccelerationZ=off  SphSenseAcceleration=off  SphSenseTorqueX=off  SphSenseTorqueY=off  SphSenseTorqueZ=off  SphSenseTorqueForce=off  SphSenseLowerLimitTorqueMag=off  SphSenseUpperLimitTorqueMag=off  SphSensingFrame=BaseFrame  SphLowerLimitSpecify=off  SphLowerLimitBound=15  SphLowerLimitBoundUnits=deg  SphLowerLimitStiffness=1e4  SphLowerLimitStiffnessUnits=N*m/deg  SphLowerLimitDamping=10  SphLowerLimitDampingUnits=N*m/(deg/s)  SphLowerLimitTransitionRegionWidth=0.1  SphLowerLimitTransitionRegionWidthUnits=deg  SphUpperLimitSpecify=off  SphUpperLimitBound=45  SphUpperLimitBoundUnits=deg  SphUpperLimitStiffness=1e4  SphUpperLimitStiffnessUnits=N*m/deg  SphUpperLimitDamping=10  SphUpperLimitDampingUnits=N*m/(deg/s)  SphUpperLimitTransitionRegionWidth=0.1  SphUpperLimitTransitionRegionWidthUnits=deg  SphPositionTargetRotationMethod=None  SphPositionTargetRotationAngleUnits=deg  SphPositionTargetRotationStandardAxis=+Z  SphPositionTargetRotationAngle=0.0  SphPositionTargetRotationArbitraryAxis=[0 0 1]  SphPositionTargetFollAlignAxisA=+X  SphPositionTargetBaseAlignAxisA=+Y  SphPositionTargetFollAlignAxisB=+Y  SphPositionTargetBaseAlignAxisB=+Z  SphPositionTargetRotationSequenceAxes=FollowerAxes  SphPositionTargetRotationSequence=XYX  SphPositionTargetRotationSequenceAngles=[0 0 0]  SphPositionTargetRotationSequenceAnglesUnits=deg  SphPositionTargetRotationMatrix=[1 0 0; 0 1 0; 0 0 1]  SphPositionTargetQuaternion=[1 0 0 0]  SphPositionTargetSpecify=off  SphPositionTargetPriority=High  SphVelocityTargetValue=[V_I0(4) V_I0(5) V_I0(6)]  SphVelocityTargetValueUnits=rad/s  SphVelocityTargetSpecify=on  SphVelocityTargetPriority=High  SphVelocityTargetInFollowerFrame=on
  Base : sm_lib/Body Elements/Brick Solid  GraphicAmbientColor=[0.15 0.15 0.15 1.0]  BasedOnType=Mass  BrickDimensions=[sc_size, sc_size, sc_size]  BrickDimensionsUnits=m  CenterOfMass=[0 0 0]  CenterOfMassUnits=m  GraphicDiffuseColor=[0.5 0.5 0.5]  Density=1000  DensityUnits=kg/m^3  DoExposeReferenceFrame=on  GraphicEmissiveColor=[0.0 0.0 0.0 1.0]  ExportEntireGeometry=off  SerializedFrames=<Frames><Frame><Id>Frame1</Id><Value><Name>F1</Name><Origin><Source>GeometricFeature</Source><FeatureName>+z surface</FeatureName></Origin><PrimaryAxis><DefinedDirection>+X</DefinedDirection><Source>ReferenceFrame</Source><SourceDirection>+X</SourceDirection><FeatureName></FeatureName></PrimaryAxis><SecondaryAxis><DefinedDirection>+Z</DefinedDirection><Source>ReferenceFrame</Source><SourceDirection>+Z</SourceDirection><FeatureName></FeatureName></SecondaryAxis></Value></Frame></Frames>  MarkerShape=Sphere  MarkerSize=10  GraphicType=FromGeometry  InertiaType=CalculateFromGeometry  Mass=m0  MassUnits=kg  MomentsOfInertia=[I0(1,1) I0(2,2) I0(3,3)]  MomentsOfInertiaUnits=kg*m^2  GraphicOpacity=1.0  ProductsOfInertia=[0 0 0]  ProductsOfInertiaUnits=kg*m^2  GraphicShininess=75  GraphicSpecularColor=[0.5 0.5 0.5 1.0]  GraphicVisPropType=SimpleVisualProperties
  Base Sensing : sm_lib/Frames and Transforms/Transform Sensor  MeasurementFrame=Base  RotationSequence=XYX  SenseAngle=off  SenseAxis=off  SenseQ=off  SenseR=on  SenseRotationSequence=off  SenseOmegaX=on  SenseOmegaY=on  SenseOmegaZ=on  SenseOmega=off  SenseQDot=off  SenseRDot=off  SenseRotationSequenceDot=off  SenseAlphaX=off  SenseAlphaY=off  SenseAlphaZ=off  SenseAlpha=off  SenseQDDot=off  SenseRDDot=off  SenseX=on  SenseY=on  SenseZ=on  SenseXYZ=off  SenseRad=off  SenseAzim=off  SenseDist=off  SenseInc=off  SenseXDot=on  SenseYDot=on  SenseZDot=on  SenseXYZDot=off  SenseRadDot=off  SenseAzimDot=off  SenseDistDot=off  SenseIncDot=off  SenseXDDot=off  SenseYDDot=off  SenseZDDot=off  SenseXYZDDot=off  SenseRadDDot=off  SenseAzimDDot=off  SenseDistDDot=off  SenseIncDDot=off
  Demux2 : Demux  Outputs=7
  Mechanism Configuration1 : sm_lib/Utilities/Mechanism Configuration  UniformGravity=Constant  GravityVector=[0 0 0]  GravityVectorUnits=m/s^2  LinearizationDelta=0.001  JointModeTransitionNonlinearIterations=2
  Mux3 : Mux  Inputs=3
  Mux4 : Mux  Inputs=6
  PS-Simulink Converter{5,8,10..15,25..26} (10 alike) : nesl_utility/PS-Simulink Converter  PhysicalDomain=network_engine_domain  SubClassName=ps_output  LeftPortType=input  RightPortType=output  PseudoPeriodic=off  Frequencies=[]  VectorFormat=1-D array  Unit=inherit  AffineConversion=off
  Simulink-PS Converter{5..11} (7 alike) : nesl_utility/Simulink-PS Converter  PhysicalDomain=network_engine_domain  SubClassName=ps_input  LeftPortType=input  RightPortType=output  PseudoPeriodic=off  Frequencies=[]  NoiseDistribution=none  NoiseParameters=[]  Unit=1  AffineConversion=off  FilteringAndDerivatives=provide  SimscapeFilterOrder=1  InputFilterTimeConstant=0.001  UdotUserProvided=0
  Solver Configuration1 : nesl_utility/Solver Configuration  PhysicalDomain=network_engine_domain  SubClassName=solver  LeftPortType=input  RightPortType=generic  Tones=[]  Harmonics=[]  SimulateNoise=off  Profile=off  UseLocalSampling=off  EnableSwitchedLinearOptims=on  FrequencyDomain=off  UseCCode=off  RelTol=0.001  AbsTol=1e-06  MinStep=1e-09  ToWorkspace=off  RevertToSquareIcSolve=off  NumHomotopyIterations=100  PhasorMode=off  PhasorModeNumHarmonics=1  ConsistencySolver=NEWTON_FTOL  IndexReductionMethod=DerivativeReplacement  DoDC=off  ResidualTolerance=1e-09  ConsistencyTolSource=GLOBAL  ConsistencyAbsTol=0.001  ConsistencyRelTol=0.001  ConsistencyTolFactor=0.001  UseLocalSolver=off  LocalSolverChoice=NE_BACKWARD_EULER_ADVANCER  ResolveIndetEquations=on  FunctionEvalNumThread=1  LocalSolverSampleTime=0.001  DoFixedCost=off  MaxNonlinIter=3  MaxModeIter=2  ComputeImpulses=off  ImpulseIterations=2  LinearAlgebra=Sparse  LinearAlgebraNumThread=0  EquationFormulation=NE_TIME_EF  DelaysMemoryBudget=1024  AutomaticFiltering=on  FilteringTimeConstant=0.001  PartitionStorageMethod=AS_NEEDED  PartitionMemoryBudget=1024  PartitionMethod=FAST  MultibodyUseLocalSolver=off  MultibodyLocalSolverChoice=ODE1  MultibodyLocalSolverSampleTime=0.001
  World Frame1 : sm_lib/Frames and Transforms/World Frame
  iiwa_joint_1_OriginTransform : sm_lib/Frames and Transforms/Rigid Transform  TranslationMethod=Cartesian  TranslationStandardOffset=0  TranslationStandardOffsetUnits=m  TranslationStandardAxis=+Z  TranslationCartesianOffset=[0, 0, 0]  TranslationCartesianOffsetUnits=m  TranslationROffset=0  TranslationROffsetUnits=m  TranslationZOffset=0  TranslationZOffsetUnits=m  TranslationThetaOffset=0  TranslationThetaOffsetUnits=deg  RotationMethod=RotationSequence  RotationAngleUnits=deg  RotationStandardAxis=+Z  RotationAngle=0.0  RotationArbitraryAxis=[0 0 1]  FollAlignAxisA=+X  BaseAlignAxisA=+Y  FollAlignAxisB=+Y  BaseAlignAxisB=+Z  RotationSequenceAxes=BaseAxes  RotationSequence=XYZ  RotationSequenceAngles=[0, 0, 0]  RotationSequenceAnglesUnits=rad  RotationMatrix=[1 0 0; 0 1 0; 0 0 1]  Quaternion=[1 0 0 0]
  joint/link 1 : Subsystem
  joint/link2 : Subsystem
  joint/link3 : Subsystem
  joint/link4 : Subsystem
  joint/link5 : Subsystem
  joint/link6 : Subsystem
  joint/link7 : Subsystem
  outputs : Subsystem
  to Homogeneous transform1 : robotcorelib/Coordinate Transformation Conversion  InputRepresentation=Rotation Matrix  InputEulerSequence=ZYX  ShowTrVecInputPort=on  OutputRepresentation=Homogeneous Transformation  OutputEulerSequence=ZYX  ShowTrVecOutputPort=on  SimulateUsing=Interpreted execution
  Conn1 : PMIOPort  Side=Left
  g_Ie : Outport
  q_m : Outport  Port=2
  q_dot_m : Outport  Port=3
  q_ddot_m : Outport  Port=4
  V : Outport  Port=5
  wires:
  PS-Simulink Converter25/1 -> to Homogeneous transform1/1
  to Homogeneous transform1/1 -> g_Ie/1
  PS-Simulink Converter5/1 -> Mux3/2
  PS-Simulink Converter8/1 -> Mux3/3
  PS-Simulink Converter26/1 -> Mux3/1
  Mux3/1 -> to Homogeneous transform1/2
  Demux2/1 -> Simulink-PS Converter5/1
  Demux2/6 -> Simulink-PS Converter10/1
  Demux2/3 -> Simulink-PS Converter7/1
  Demux2/2 -> Simulink-PS Converter6/1  "f_elbow"
  Demux2/5 -> Simulink-PS Converter9/1
  Demux2/7 -> Simulink-PS Converter11/1
  outputs/3(q_ddot_m) -> q_ddot_m/1
  f_m/1 -> Demux2/1
  Demux2/4 -> Simulink-PS Converter8/1
  outputs/2(q_dot_m) -> q_dot_m/1
  outputs/1(q_m) -> q_m/1
  PS-Simulink Converter13/1 -> Mux4/4  "wx"
  PS-Simulink Converter12/1 -> Mux4/3  "vz"
  PS-Simulink Converter10/1 -> Mux4/1  "vx"
  Mux4/1 -> V/1
  PS-Simulink Converter11/1 -> Mux4/2  "vy"
  PS-Simulink Converter14/1 -> Mux4/5  "wy"
  PS-Simulink Converter15/1 -> Mux4/6  "wz"
  connections:
  Base Sensing/LConn1 -- Conn1/RConn1 -- Mechanism Configuration1/RConn1 -- World Frame1/RConn1 -- 6-DOF Joint/LConn1 -- Solver Configuration1/RConn1
  Base Sensing/RConn1 -- Base/RConn1 -- 6-DOF Joint/RConn1
  Base Sensing/RConn6 -- PS-Simulink Converter26/LConn1
  Base Sensing/RConn8 -- PS-Simulink Converter8/LConn1
  Base Sensing/RConn2 -- PS-Simulink Converter25/LConn1
  Base Sensing/RConn7 -- PS-Simulink Converter5/LConn1
  iiwa_joint_1_OriginTransform/RConn1 -- joint/link 1/LConn1
  joint/link3/RConn3 -- outputs/LConn10
  joint/link5/RConn3 -- outputs/LConn12
  Simulink-PS Converter9/RConn1 -- joint/link5/LConn2
  joint/link4/LConn1 -- joint/link3/RConn1
  joint/link4/RConn3 -- outputs/LConn11
  joint/link5/RConn4 -- outputs/LConn19
  Simulink-PS Converter10/RConn1 -- joint/link6/LConn2
  joint/link5/LConn1 -- joint/link4/RConn1
  joint/link7/RConn5 -- outputs/LConn21
  joint/link2/RConn4 -- outputs/LConn16
  joint/link 1/LConn2 -- Simulink-PS Converter5/RConn1
  outputs/LConn1 -- joint/link 1/RConn2
  joint/link5/RConn2 -- outputs/LConn5
  joint/link7/RConn3 -- outputs/LConn7
  joint/link7/RConn4 -- outputs/LConn14
  joint/link2/RConn2 -- outputs/LConn2
  Simulink-PS Converter11/RConn1 -- joint/link7/LConn2
  joint/link 1/RConn3 -- outputs/LConn8
  Simulink-PS Converter7/RConn1 -- joint/link3/LConn2
  joint/link6/LConn1 -- joint/link5/RConn1
  joint/link2/RConn3 -- outputs/LConn9
  joint/link 1/RConn4 -- outputs/LConn15
  Simulink-PS Converter6/RConn1 -- joint/link2/LConn2
  joint/link3/LConn1 -- joint/link2/RConn1
  joint/link4/RConn2 -- outputs/LConn4
  joint/link6/RConn2 -- outputs/LConn6
  joint/link4/RConn4 -- outputs/LConn18
  joint/link3/RConn2 -- outputs/LConn3
  joint/link6/RConn3 -- outputs/LConn13
  Simulink-PS Converter8/RConn1 -- joint/link4/LConn2
  joint/link6/RConn4 -- outputs/LConn20
  joint/link3/RConn4 -- outputs/LConn17
  joint/link7/LConn1 -- joint/link6/RConn1
  joint/link 1/RConn1 -- joint/link2/LConn1
  Base/LConn1 -- iiwa_joint_1_OriginTransform/LConn1
  Base Sensing/RConn9 -- PS-Simulink Converter10/LConn1
  Base Sensing/RConn10 -- PS-Simulink Converter11/LConn1
  Base Sensing/RConn11 -- PS-Simulink Converter12/LConn1
  Base Sensing/RConn3 -- PS-Simulink Converter13/LConn1
  Base Sensing/RConn4 -- PS-Simulink Converter14/LConn1
  Base Sensing/RConn5 -- PS-Simulink Converter15/LConn1
